simulink model "sim"  (R2019b)
settings: Solver=VariableStepAuto  StartTime=0.0  StopTime=10.0  RelTol=1e-3
undefined symbols (not defined in the file or in its folder): get, hot
libraries: visionsources x2, dspsnks4 x1
settings Model: Creator=vardhan  LastModifiedBy=vardhan

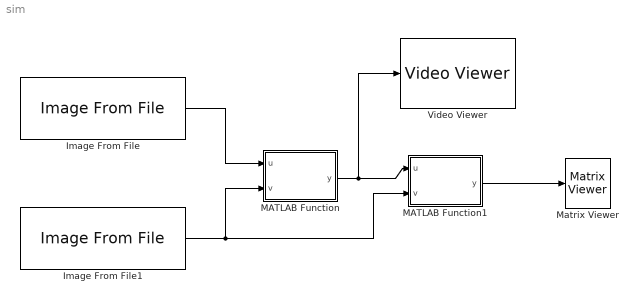
== system sim ==
  Image From File : visionsources/Image From File  Tag=vipblks_nd  FileName=C:\Users\vardhan\Downloads\DSP project\a.png  Ts=inf  imagePorts=One multidimensional signal  OutPortLabels=R|G|B  ImageDataType=Inherit from input image  sdImageDataType=uint(8)  Signed=on  WordLength=16  FractionLengthMode=User-defined  FractionLength=15
      settings: SourceProductName=Computer Vision Toolbox
  Image From File1 : visionsources/Image From File  Tag=vipblks_nd  FileName=C:\Users\vardhan\Downloads\DSP project\cameraman.tif  Ts=inf  imagePorts=One multidimensional signal  OutPortLabels=R|G|B  ImageDataType=Inherit from input image  sdImageDataType=uint(8)  Signed=on  WordLength=16  FractionLengthMode=User-defined  FractionLength=15
      settings: SourceProductName=Computer Vision Toolbox
  MATLAB Function : MATLAB Function  TreatAsAtomicUnit=on
  MATLAB Function1 : MATLAB Function  TreatAsAtomicUnit=on
  Matrix Viewer : dspsnks4/Matrix Viewer  ImageParams=off  CMapStr=hot(256)  AxisColorbar=on  AxisParams=off  AxisOrigin=Upper left corner  AxisTickMode=Auto  XTickRange=[0 1]  YTickRange=[0 1]  XLabel=X-axis  YLabel=Y-axis  ZLabel=Z-axis  FigPos=get(0,'defaultfigureposition')  AxisZoom=off
      settings: SourceProductName=DSP System Toolbox  SourceProductBaseCode=DS  YMin=-1.0  YMax=1.0
  Video Viewer : VideoViewer  FigPos=[474 535 418 304]
  wires:
  Image From File/1 -> MATLAB Function/1(u)
  Image From File1/1 -> MATLAB Function1/2(v), MATLAB Function/2(v)
  MATLAB Function/1(y) -> MATLAB Function1/1(u), Video Viewer/1
  MATLAB Function1/1(y) -> Matrix Viewer/1

== matlab function sim/MATLAB Function1 ==
  data: u input; y output; v input
function y = fcn(u,v)
coder.extrinsic('dct2');
coder.extrinsic('idct2');
dct_a = zeros(256,256);
dct_b = zeros(256,256);
c = zeros(256,256);
p = zeros(256,256);

dct_a = dct2(u);
dct_b = dct2(v);
c = dct_a - dct_b;

p = uint8(255 * c);
p = p(1:128,1:128);

y = p;

== matlab function sim/MATLAB Function ==
  data: u input; v input; y output
function y = fcn(u,v)
coder.extrinsic('dct2');
coder.extrinsic('idct2');
dct_b = zeros(256,256);
idct_sum = zeros(256,256);
sum = zeros(256,256);

ba = imbinarize(u); % conversion of image into binary
[m,n]=size(ba);
a1 = [ba, zeros(256-m,256-n);zeros(256-m,256)]; % zero padding
dct_b = dct2(v);
sum = double(a1) + dct_b; % addition of two images
idct_sum = idct2(sum);
idct_sum = uint8(idct_sum);

%Error using imwrite (line 528)
%Unable to open file "hidden_img.png" for writing. You might not have
%write permission.
%Error in hideimg (line 19)
%imwrite(double(idct_sum),'hidden_img.png');

y = idct_sum;
